simulink model "Liver_Insulin35"  (R2018a)
settings: Solver=VariableStepAuto  StartTime=0.0  StopTime=10.0  RelTol=1e-3
undefined symbols (not defined in the file): Q_i_A, Q_i_G, Q_i_L, V_i_L
settings Model: Creator=cgonterman  LastModifiedBy=cgonterman

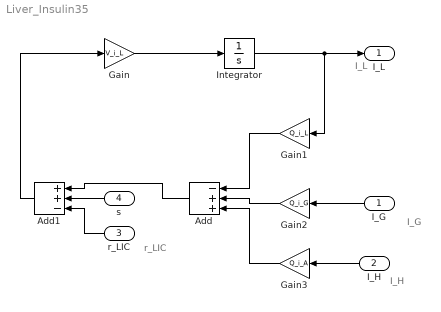
== system Liver_Insulin35 ==
  note: r_LIC
  note: I_H
  note: I_G
  note: I_L
  "I_G " : Inport
  "I_H " : Inport  Port=2
  "r_LIC " : Inport  Port=3
  "s " : Inport  Port=4
  Add : Sum  Inputs=-++
  Add1 : Sum  Inputs=++-
  Gain : Gain  Gain=V_i_L
  Gain1 : Gain  Gain=Q_i_L
  Gain2 : Gain  Gain=Q_i_G
  Gain3 : Gain  Gain=Q_i_A
  Integrator : Integrator
  "I_L " : Outport
  wires:
  "I_G "/1 -> Gain2/1
  "I_H "/1 -> Gain3/1
  Gain2/1 -> Add/2
  Gain3/1 -> Add/3
  Gain1/1 -> Add/1
  "r_LIC "/1 -> Add1/3
  "s "/1 -> Add1/2
  Add/1 -> Add1/1
  Add1/1 -> Gain/1
  Gain/1 -> Integrator/1
  Integrator/1 -> Gain1/1, "I_L "/1
